simulink model "lupacchiotti_simulink"  (R2024b)
settings: Solver=VariableStepAuto  StartTime=0.0  StopTime=1.0  RelTol=1e-3
values from neighbouring files (symbols this model uses):
  C = [1, 0]    [lupacchiotti.m]
  Cm_e = (k * theta_e) / tau(theta_e)    [lupacchiotti.m]
  W = 1.5    [lupacchiotti.m]
  x1_e = theta_e    [lupacchiotti.m]
  x2_e = 0    [lupacchiotti.m]
libraries: cstblocks x1
settings Model: Creator=User  LastModifiedBy=fippo

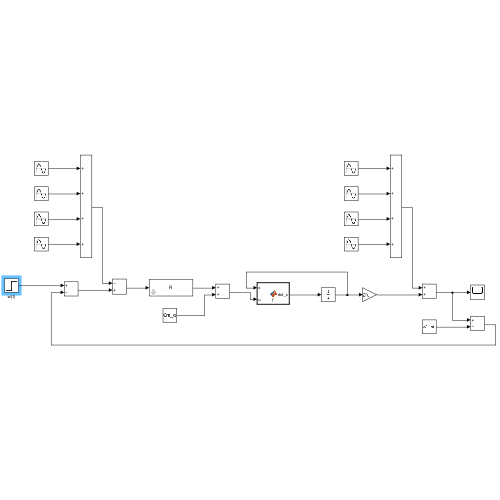
[thumbnail: Simulink's stored preview of the top-level diagram]
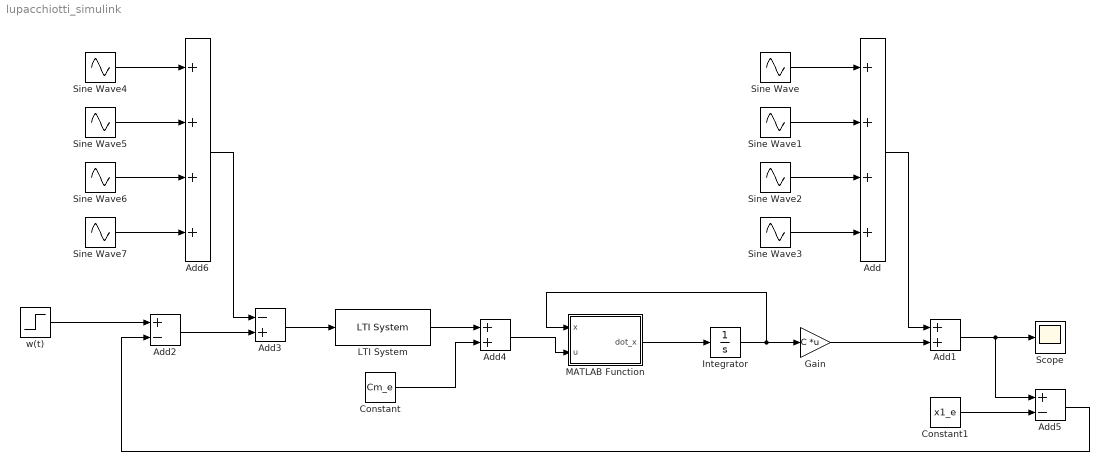
== system lupacchiotti_simulink ==
  Add : Sum  Inputs=++++
  Add1 : Sum
  Add2 : Sum  Inputs=+-
  Add3 : Sum  Inputs=-+
  Add4 : Sum
  Add5 : Sum  Inputs=+-
  Add6 : Sum  Inputs=++++
  Constant : Constant  Value=Cm_e
  Constant1 : Constant  Value=x1_e
  Gain : Gain  Gain=C  Multiplication=Matrix(K*u)
  Integrator : Integrator  InitialCondition=[x1_e; x2_e]
  LTI System : cstblocks/LTI System  sys=R  IC=[]  PadeOrder=0
  MATLAB Function : MATLAB Function  TreatAsAtomicUnit=on
  Scope : Scope
  Sine Wave : Sin  Amplitude=0.2  Frequency=0.1*1  SampleTime=0
  Sine Wave1 : Sin  Amplitude=0.2  Frequency=0.1*2  SampleTime=0
  Sine Wave2 : Sin  Amplitude=0.2  Frequency=0.1*3  SampleTime=0
  Sine Wave3 : Sin  Amplitude=0.2  Frequency=0.1*4  SampleTime=0
  Sine Wave4 : Sin  Amplitude=0.2  Frequency=2*10^5*1  SampleTime=0
  Sine Wave5 : Sin  Amplitude=0.2  Frequency=2*10^5*2  SampleTime=0
  Sine Wave6 : Sin  Amplitude=0.2  Frequency=2*10^5*3  SampleTime=0
  Sine Wave7 : Sin  Amplitude=0.2  Frequency=2*10^5*4  SampleTime=0
  w(t) : Step  After=W  SampleTime=0
  wires:
  w(t)/1 -> Add2/1
  Add2/1 -> Add3/2
  Add3/1 -> LTI System/1
  LTI System/1 -> Add4/1
  Constant/1 -> Add4/2
  Add4/1 -> MATLAB Function/2(u)
  MATLAB Function/1(dot_x) -> Integrator/1
  Integrator/1 -> MATLAB Function/1(x), Gain/1
  Gain/1 -> Add1/2
  Add1/1 -> Scope/1, Add5/1
  Constant1/1 -> Add5/2
  Add5/1 -> Add2/2
  Sine Wave3/1 -> Add/4
  Sine Wave2/1 -> Add/3
  Sine Wave1/1 -> Add/2
  Sine Wave/1 -> Add/1
  Add/1 -> Add1/1
  Sine Wave5/1 -> Add6/2
  Sine Wave4/1 -> Add6/1
  Sine Wave6/1 -> Add6/3
  Sine Wave7/1 -> Add6/4
  Add6/1 -> Add3/1

== matlab function lupacchiotti_simulink/MATLAB Function ==
  data: x input; u input; dot_x output
function dot_x = f(x, u)

k     = 500;        % [N/m^2]
beta  = 0.5;        % [N*s/m^2]
alpha = deg2rad(50);% [rad]
J     = 400;        % [J*m^2]

dot_x = zeros(2,1);

dot_x(1) = x(2);

dot_x(2) = (u*cos(alpha)/(1-sin(alpha)*cos(x(1)^2)) - beta*x(2) -k*x(1))/J;
